simulink model "prach_shortFormat_fftShift"  (R2023b)
settings: Solver=FixedStepDiscrete  StartTime=0.0  StopTime=prach_short.SimulationTime  FixedStep=1  RelTol=1e-3  EnableMultiTasking=on
PreLoadFcn:
  | warning off Simulink:Commands:SetParamLinkChangeWarn
  | warning off Simulink:Commands:LoadMdlParameterizedLink
  | warning off Simulink:SL_SetParamLinkChangeWarn
  | warning off Simulink:SL_LoadMdlParameterizedLink
  | setup_prach_shortFormat;
InitFcn:
  | setup_prach_shortFormat;
StopFcn:
  | prach_post_run_script
values from neighbouring files (symbols this model uses):
  ConfigTable = [16 1 9,20,20,20,20,20,20,20,20,20 0 2 6 2 4 ... (first row only)    [ConfigIndexTable.m]
  NTxAnts = 4    [setup_prach_shortFormat.m]    (also in setup_prach_shortFormat_fftShift.m)
undefined symbols (not defined in the file or in its folder): AdvDSPBChannelOutDisplay, AdvDSPBDMemDisplay, BW, ControlDecode, display, dpoly, dspba, dspba_ChannelInVis, dspba_ChannelOutVis, dspba_internal_get_channel_ports, evalAionMaskParam, latency, PRACH_CC, PRACH_regs, prach_short, PrachLib, PrachLib_FFTshift, primtype, RemoveCP, Stream2BlockConv, UseDontCare, value, waveconfig
libraries: DSPBAPrim x397, DSPBAControl x16, DSPBAModelBus x7, DSPBABase x5, DSPBAUtilities x5, simulink x2, DSPBAVectorUtil x1, DspbAdvFftLibrary x1
(part 1 of 5)
Description:
  | This design Implements a PRACH detection for short format for TDD configurations.
settings Model: Creator=lrigby  LastModifiedBy=5g
settings SolverCC: AlgebraicLoopSolver=TrustRegion
settings DataIOCC: LimitDataPoints=on  SaveFormat=StructureWithTime  SignalLoggingSaveFormat=ModelDataLogs  ReturnWorkspaceOutputs=off
settings OptimizationCC: ExpressionDepthLimit=2147483647  InitFltsAndDblsToZero=on  LifeSpan=inf
settings DebuggingCC: SaveWithParameterizedLinksMsg=none  UnderspecifiedInitializationDetection=Classic  MergeDetectMultiDrivingBlocksExec=none  SignalResolutionControl=TryResolveAllWithWarning  SolverPrmCheckMsg=warning  ParameterPrecisionLossMsg=none  UnconnectedInputMsg=warning  UnconnectedOutputMsg=warning  UnconnectedLineMsg=warning  StateNameClashWarn=warning  SFUnexpectedBacktrackingDiag=warning  SFNoUnconditionalDefaultTransitionDiag=warning  SFExecutionAtInitializationDiag=none  ArithmeticOperatorsInVariantConditions=warning
settings HardwareCC: ProdBitPerPointer=32  ProdBitPerSizeT=32  ProdBitPerPtrDiffT=32  ProdLargestAtomicFloat=None  ProdIntDivRoundTo=Undefined  ProdEndianess=Unspecified  ProdWordSize=32  ProdHWDeviceType=ASIC/FPGA  TargetBitPerLong=64  TargetBitPerPointer=64  TargetBitPerSizeT=64  TargetBitPerPtrDiffT=64  TargetLongLongMode=on  TargetIntDivRoundTo=Zero  TargetEndianess=LittleEndian  TargetWordSize=64  TargetHWDeviceType=MATLAB Host  ProdEqTarget=off
settings ModelReferenceCC: EnableRefExpFcnMdlSchedulingChecks=on  PropagateSignalLabelsOutOfModel=off
settings SFSimCC: SimUseLocalCustomCode=off  SimParseCustomCode=off  CustomCodeUndefinedFunction=UseInterfaceOnly
settings RTWCC: RTWUseLocalCustomCode=off  DLArmComputeVersion=19.05
settings CodeAppCC: StateflowObjectComments=on
settings GRTTargetCC: TargetFcnLib=ansi_tfl_tmw.mat  TargetLangStandard=C89/C90 (ANSI)  CombineOutputUpdateFcns=off  GRTInterface=on
settings ConfigComp: CovMetricSettings=dw  CovSaveCumulativeToWorkspaceVar=on  CovSaveSingleToWorkspaceVar=on  CovExternalEMLEnable=off  CovSFcnEnable=off

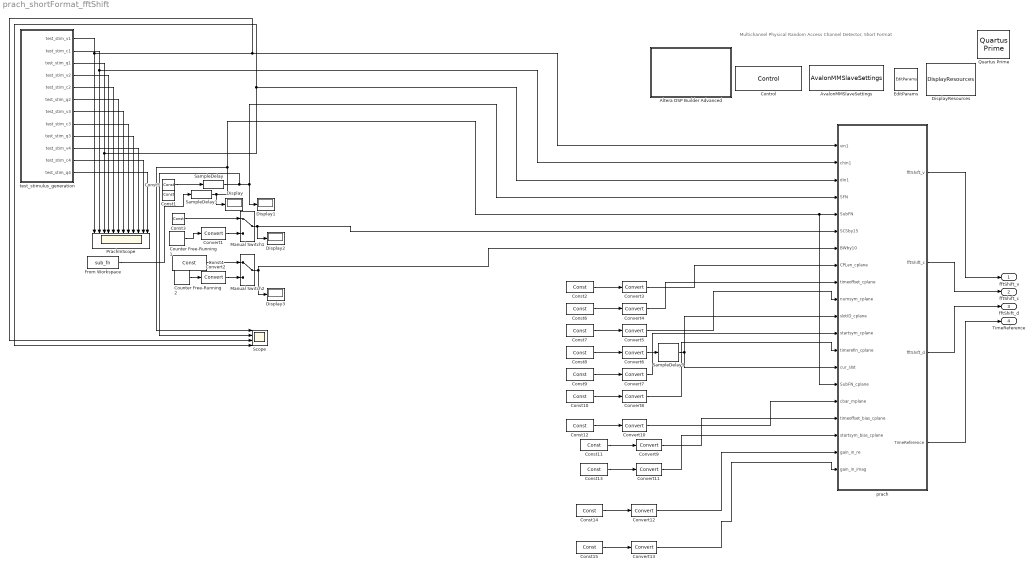
== system prach_shortFormat_fftShift ==
  note: Multichannel Physical Random
      | Access Channel Detector, Short Format
  Altera DSP Builder Advanced : Subsystem  mask(DSP Builder Advanced Blockset Ignored Block){}
      settings: OpenFcn=web('http://www.altera.com', '-new');
      mask Display: image(imread('alteralogo.tif'));
  AvalonMMSlaveSettings : DSPBABase/AvalonMMSlaveSettings
  Const1 : DSPBAPrim/Const  primtype=const  nInputs=0  nOutputs=1  omode=Specify via dialog  otype=uint(8)  scale=2^-0  rndmethod=Unbiased  factor=1  satmethod=Symmetric  shift_vec=[0 1 2 -1]  value=SubF  inPortNames=['+'; '+';]  outPortNames=[' ']  dspbaimage=dspba_prim.svg  text=fprintf('%s', num2str(value));  style=Optimised  visibilities=8 + 1024  floatPrecision=float32_m23  warnSaturation=on  version=20211007  SampleTime=inf
  Const{2,9..10,12..13,15} (6 alike) : DSPBAPrim/Const  primtype=const  nInputs=0  nOutputs=1  omode=Inherit via internal rule  otype=ufix(23)  scale=1  rndmethod=Unbiased  factor=1  satmethod=Symmetric  shift_vec=[0 1 2 -1]  value=0  inPortNames=['+'; '+';]  outPortNames=[' ']  dspbaimage=dspba_prim.svg  text=fprintf('%s', num2str(value));  style=Optimised  visibilities=8 + 1024  floatPrecision=float32_m23  warnSaturation=on  version=20211007  SampleTime=inf
  Const11 : DSPBAPrim/Const  primtype=const  nInputs=0  nOutputs=1  omode=Inherit via internal rule  otype=ufix(23)  scale=1  rndmethod=Unbiased  factor=1  satmethod=Symmetric  shift_vec=[0 1 2 -1]  value=220  inPortNames=['+'; '+';]  outPortNames=[' ']  dspbaimage=dspba_prim.svg  text=fprintf('%s', num2str(value));  style=Optimised  visibilities=8 + 1024  floatPrecision=float32_m23  warnSaturation=on  version=20211007  SampleTime=inf
  Const14 : DSPBAPrim/Const  primtype=const  nInputs=0  nOutputs=1  omode=Inherit via internal rule  otype=ufix(23)  scale=1  rndmethod=Unbiased  factor=1  satmethod=Symmetric  shift_vec=[0 1 2 -1]  value=1  inPortNames=['+'; '+';]  outPortNames=[' ']  dspbaimage=dspba_prim.svg  text=fprintf('%s', num2str(value));  style=Optimised  visibilities=8 + 1024  floatPrecision=float32_m23  warnSaturation=on  version=20211007  SampleTime=inf
  Const3 : DSPBAPrim/Const  primtype=const  nInputs=0  nOutputs=1  omode=Specify via dialog  otype=uint(2)  scale=1  rndmethod=Unbiased  factor=1  satmethod=Symmetric  shift_vec=[0 1 2 -1]  value=floor(waveconfig.PRACH.Config.SubcarrierSpacing/15)  inPortNames=['+'; '+';]  outPortNames=[' ']  dspbaimage=dspba_prim.svg  text=fprintf('%s', num2str(value));  style=Optimised  visibilities=8 + 1024  floatPrecision=float32_m23  warnSaturation=on  version=20211007  SampleTime=inf
  Const4 : DSPBAPrim/Const  primtype=const  nInputs=0  nOutputs=1  omode=Specify via dialog  otype=uint(4)  scale=1  rndmethod=Unbiased  factor=1  satmethod=Symmetric  shift_vec=[0 1 2 -1]  value=floor(BW/10)  inPortNames=['+'; '+';]  outPortNames=[' ']  dspbaimage=dspba_prim.svg  text=fprintf('%s', num2str(value));  style=Optimised  visibilities=8 + 1024  floatPrecision=float32_m23  warnSaturation=on  version=20211007  SampleTime=inf
  Const5 : DSPBAPrim/Const  primtype=const  nInputs=0  nOutputs=1  omode=Specify via dialog  otype=uint(12)  scale=2^-0  rndmethod=Unbiased  factor=1  satmethod=Symmetric  shift_vec=[0 1 2 -1]  value=SFN  inPortNames=['+'; '+';]  outPortNames=[' ']  dspbaimage=dspba_prim.svg  text=fprintf('%s', num2str(value));  style=Optimised  visibilities=8 + 1024  floatPrecision=float32_m23  warnSaturation=on  version=20211007  SampleTime=inf
  Const6 : DSPBAPrim/Const  primtype=const  nInputs=0  nOutputs=1  omode=Inherit via internal rule  otype=ufix(23)  scale=1  rndmethod=Unbiased  factor=1  satmethod=Symmetric  shift_vec=[0 1 2 -1]  value=1156  inPortNames=['+'; '+';]  outPortNames=[' ']  dspbaimage=dspba_prim.svg  text=fprintf('%s', num2str(value));  style=Optimised  visibilities=8 + 1024  floatPrecision=float32_m23  warnSaturation=on  version=20211007  SampleTime=inf
  Const7 : DSPBAPrim/Const  primtype=const  nInputs=0  nOutputs=1  omode=Inherit via internal rule  otype=ufix(23)  scale=1  rndmethod=Unbiased  factor=1  satmethod=Symmetric  shift_vec=[0 1 2 -1]  value=12  inPortNames=['+'; '+';]  outPortNames=[' ']  dspbaimage=dspba_prim.svg  text=fprintf('%s', num2str(value));  style=Optimised  visibilities=8 + 1024  floatPrecision=float32_m23  warnSaturation=on  version=20211007  SampleTime=inf
  Const8 : DSPBAPrim/Const  primtype=const  nInputs=0  nOutputs=1  omode=Inherit via internal rule  otype=ufix(23)  scale=1  rndmethod=Unbiased  factor=1  satmethod=Symmetric  shift_vec=[0 1 2 -1]  value=1  inPortNames=['+'; '+';]  outPortNames=[' ']  dspbaimage=dspba_prim.svg  text=fprintf('%s', num2str(value));  style=Optimised  visibilities=8 + 1024  floatPrecision=float32_m23  warnSaturation=on  version=20211007  SampleTime=inf
  Control : DSPBABase/Control  generate=on  language=VHDL  destination=./rtl  make_full_path=off  path_is_relative=on  autotestbench=on  signaldepth=2  coveragetestbench=off  logs=off  spacewidth=2  spacenum=1  addrwidth=10  datawidth=16  dataendian=Big Endian  hierarchicalnames=on  ramThresholdBits=-1  distRamThresholdBits=-1  mlabThresholdBits=-1  hardMultiplierThresholdLuts=-1  version=20090407  errorOnChanMismatch=1  errorOnGPIOMismatch=0  importModelsimResults=0  cycleAccurate=off  reinterpretCastMult=off  paramFile=prach_shortFormat_fftShift_params.xml
  Convert1 : DSPBAPrim/Convert  primtype=convert  nInputs=1  nOutputs=1  omode=Specify via dialog  otype=uint(2)  scale=1  rndmethod=Biased  factor=1  satmethod=None  shift_vec=[0 1 2 -1]  value=round([0:255]/17)  inPortNames=[' '; ' ';]  outPortNames=[' '; 'c']  dspbaimage=dspba_prim_wide.svg  text=fprintf('convert');  style=Optimised  visibilities=8+64+256+2^17  clipdetect=off  floatPrecision=float32_m23  advOptions=[]  version=20211007
  Convert10 : DSPBAPrim/Convert  primtype=convert  nInputs=1  nOutputs=1  omode=boolean  otype=ufix(2)  scale=1  rndmethod=Biased  factor=1  satmethod=None  shift_vec=[0 1 2 -1]  value=round([0:255]/17)  inPortNames=[' '; ' ';]  outPortNames=[' '; 'c']  dspbaimage=dspba_prim_wide.svg  text=fprintf('convert');  style=Optimised  visibilities=8+64+256+2^17  clipdetect=off  floatPrecision=float32_m23  advOptions=[]  version=20211007
  Convert{3..4,9,11} (4 alike) : DSPBAPrim/Convert  primtype=convert  nInputs=1  nOutputs=1  omode=Specify via dialog  otype=ufix(23)  scale=1  rndmethod=Biased  factor=1  satmethod=None  shift_vec=[0 1 2 -1]  value=round([0:255]/17)  inPortNames=[' '; ' ';]  outPortNames=[' '; 'c']  dspbaimage=dspba_prim_wide.svg  text=fprintf('convert');  style=Optimised  visibilities=8+64+256+2^17  clipdetect=off  floatPrecision=float32_m23  advOptions=[]  version=20211007
  Convert12 : DSPBAPrim/Convert  primtype=convert  nInputs=1  nOutputs=1  omode=Specify via dialog  otype=fixdt(0,16,14)  scale=0  rndmethod=Biased  factor=1  satmethod=None  shift_vec=[0 1 2 -1]  value=round([0:255]/17)  inPortNames=[' '; ' ';]  outPortNames=[' '; 'c']  dspbaimage=dspba_prim_wide.svg  text=fprintf('convert');  style=Optimised  visibilities=8+64+256+2^17  clipdetect=off  floatPrecision=float32_m23  advOptions=[]  version=20211007
  Convert13 : DSPBAPrim/Convert  primtype=convert  nInputs=1  nOutputs=1  omode=Specify via dialog  otype=fixdt(0,16,14)  scale=0  rndmethod=Biased  factor=1  satmethod=None  shift_vec=[0 1 2 -1]  value=round([0:255]/17)  inPortNames=[' '; ' ';]  outPortNames=[' '; 'c']  dspbaimage=dspba_prim_wide.svg  text=fprintf('convert');  style=Optimised  visibilities=8+64+256+2^17  clipdetect=off  floatPrecision=float32_m23  advOptions=[]  version=20211007
  Convert2 : DSPBAPrim/Convert  primtype=convert  nInputs=1  nOutputs=1  omode=Specify via dialog  otype=uint(8)  scale=1  rndmethod=Biased  factor=1  satmethod=None  shift_vec=[0 1 2 -1]  value=round([0:255]/17)  inPortNames=[' '; ' ';]  outPortNames=[' '; 'c']  dspbaimage=dspba_prim_wide.svg  text=fprintf('convert');  style=Optimised  visibilities=8+64+256+2^17  clipdetect=off  floatPrecision=float32_m23  advOptions=[]  version=20211007
  Convert5 : DSPBAPrim/Convert  primtype=convert  nInputs=1  nOutputs=1  omode=Specify via dialog  otype=ufix(4)  scale=1  rndmethod=Biased  factor=1  satmethod=None  shift_vec=[0 1 2 -1]  value=round([0:255]/17)  inPortNames=[' '; ' ';]  outPortNames=[' '; 'c']  dspbaimage=dspba_prim_wide.svg  text=fprintf('convert');  style=Optimised  visibilities=8+64+256+2^17  clipdetect=off  floatPrecision=float32_m23  advOptions=[]  version=20211007
  Convert6 : DSPBAPrim/Convert  primtype=convert  nInputs=1  nOutputs=1  omode=Specify via dialog  otype=ufix(2)  scale=1  rndmethod=Biased  factor=1  satmethod=None  shift_vec=[0 1 2 -1]  value=round([0:255]/17)  inPortNames=[' '; ' ';]  outPortNames=[' '; 'c']  dspbaimage=dspba_prim_wide.svg  text=fprintf('convert');  style=Optimised  visibilities=8+64+256+2^17  clipdetect=off  floatPrecision=float32_m23  advOptions=[]  version=20211007
  Convert7 : DSPBAPrim/Convert  primtype=convert  nInputs=1  nOutputs=1  omode=Specify via dialog  otype=ufix(4)  scale=1  rndmethod=Biased  factor=1  satmethod=None  shift_vec=[0 1 2 -1]  value=round([0:255]/17)  inPortNames=[' '; ' ';]  outPortNames=[' '; 'c']  dspbaimage=dspba_prim_wide.svg  text=fprintf('convert');  style=Optimised  visibilities=8+64+256+2^17  clipdetect=off  floatPrecision=float32_m23  advOptions=[]  version=20211007
  Convert8 : DSPBAPrim/Convert  primtype=convert  nInputs=1  nOutputs=1  omode=Specify via dialog  otype=ufix(29)  scale=1  rndmethod=Biased  factor=1  satmethod=None  shift_vec=[0 1 2 -1]  value=round([0:255]/17)  inPortNames=[' '; ' ';]  outPortNames=[' '; 'c']  dspbaimage=dspba_prim_wide.svg  text=fprintf('convert');  style=Optimised  visibilities=8+64+256+2^17  clipdetect=off  floatPrecision=float32_m23  advOptions=[]  version=20211007
  Counter Free-Running1 : simulink/Sources/Counter Free-Running  NumBits=2  tsamp=-1
  Counter Free-Running2 : simulink/Sources/Counter Free-Running  NumBits=4  tsamp=-1
  Display{,1..3} (4 alike) : Display
  DisplayResources : DSPBAUtilities/DisplayResources  mults=0  luts=0  memorybits=0
  EditParams : DSPBABase/EditParams  version=20090407
  From Workspace : FromWorkspace  VariableName=sub_fn  OutDataTypeStr=uint8  SampleTime=prach_short.SampleTime  OutputAfterFinalValue=Setting to zero
  Manual Switch1 : ManualSwitch
  Manual Switch2 : ManualSwitch
  PrachInScope : Scope  NumInputPorts=12
  Quartus Prime : DSPBABase/Quartus Prime  version=20090407
  SampleDelay : DSPBAPrim/SampleDelay  primtype=sampdelay  nInputs=1  nOutputs=1  omode=Inherit via internal rule  otype=sfix(16)  scale=2^-15  rndmethod=Unbiased  factor=1  satmethod=Symmetric  shift_vec=[0 1 2 -1]  floatPrecision=float32_m23  value=0  inPortNames=[' '; ' ';]  outPortNames=[' ']  dspbaimage=dspba_prim.svg  text=dpoly(1, eye(1,value+1), 'z')  style=Optimised  visibilities=8 + 1024 + 2^17 + 2^18  flexible=off  slackgroup=0  augmented=0  version=20211007  advOptions=[]
  SampleDelay1 : DSPBAPrim/SampleDelay  primtype=sampdelay  nInputs=1  nOutputs=1  omode=Inherit via internal rule  otype=sfix(16)  scale=2^-15  rndmethod=Unbiased  factor=1  satmethod=Symmetric  shift_vec=[0 1 2 -1]  floatPrecision=float32_m23  value=0  inPortNames=[' '; ' ';]  outPortNames=[' ']  dspbaimage=dspba_prim.svg  text=dpoly(1, eye(1,value+1), 'z')  style=Optimised  visibilities=8 + 1024 + 2^17 + 2^18  flexible=off  slackgroup=0  augmented=0  version=20211007  advOptions=[]
  SampleDelay5 : DSPBAPrim/SampleDelay  primtype=sampdelay  nInputs=1  nOutputs=1  omode=Inherit via internal rule  otype=sfix(16)  scale=2^-15  rndmethod=Unbiased  factor=1  satmethod=Symmetric  shift_vec=[0 1 2 -1]  floatPrecision=float32_m23  value=1  inPortNames=[' '; ' ';]  outPortNames=[' ']  dspbaimage=dspba_prim.svg  text=dpoly(1, eye(1,value+1), 'z')  style=Optimised  visibilities=8 + 1024 + 2^17 + 2^18  flexible=off  slackgroup=0  augmented=0  version=20211007  advOptions=[]
  Scope : Scope  NumInputPorts=4
  prach : Subsystem
  test_stimulus_generation : Subsystem
  fftShift_v : Outport
  fftShift_c : Outport  Port=2
  fftShift_d : Outport  Port=3
  TimeReference : Outport  Port=4
  wires:
  test_stimulus_generation/2(test_stim_c1) -> PrachInScope/2, prach/2(chin1)
  test_stimulus_generation/3(test_stim_q1) -> PrachInScope/3, Scope/4, prach/3(din1)
  test_stimulus_generation/4(test_stim_v2) -> PrachInScope/4
  test_stimulus_generation/5(test_stim_c2) -> PrachInScope/5
  test_stimulus_generation/6(test_stim_q2) -> PrachInScope/6
  test_stimulus_generation/7(test_stim_v3) -> PrachInScope/7
  test_stimulus_generation/8(test_stim_c3) -> PrachInScope/8
  test_stimulus_generation/9(test_stim_q3) -> PrachInScope/9
  test_stimulus_generation/10(test_stim_v4) -> PrachInScope/10
  test_stimulus_generation/11(test_stim_c4) -> PrachInScope/11
  test_stimulus_generation/12(test_stim_q4) -> PrachInScope/12
  test_stimulus_generation/1(test_stim_v1) -> PrachInScope/1, Scope/3, prach/1(vin1)
  Const5/1 -> SampleDelay/1
  From Workspace/1 -> SampleDelay1/1
  Const3/1 -> Manual Switch1/1
  Const4/1 -> Manual Switch2/1
  Manual Switch1/1 -> prach/6(SCSby15), Display2/1
  Manual Switch2/1 -> prach/7(BWby10), Display3/1
  Counter Free-Running1/1 -> Convert1/1
  Convert1/1 -> Manual Switch1/2
  Counter Free-Running2/1 -> Convert2/1
  Convert2/1 -> Manual Switch2/2
  SampleDelay/1 -> Scope/2, Display1/1, prach/4(SFN)
  SampleDelay1/1 -> Display/1, Scope/1, prach/15(SubFN_cplane), prach/5(SubFN)
  prach/3(fftShift_d) -> fftShift_d/1
  prach/2(fftShift_c) -> fftShift_c/1
  prach/4(TimeReference) -> TimeReference/1
  prach/1(fftShift_v) -> fftShift_v/1
  Const11/1 -> Convert9/1
  Convert9/1 -> prach/17(timeoffset_bias_cplane)
  Convert4/1 -> prach/9(timeoffset_cplane)
  Const8/1 -> Convert6/1
  Const10/1 -> Convert8/1
  Convert3/1 -> prach/8(CPLen_cplane)
  Const15/1 -> Convert13/1
  Const12/1 -> Convert10/1
  Convert5/1 -> prach/10(numsym_cplane)
  Const6/1 -> Convert4/1
  Convert7/1 -> prach/12(startsym_cplane)
  Convert8/1 -> prach/13(timerefin_cplane)
  Const7/1 -> Convert5/1
  Const2/1 -> Convert3/1
  Const9/1 -> Convert7/1
  Convert13/1 -> prach/20(gain_in_imag)
  Const13/1 -> Convert11/1
  Convert12/1 -> prach/19(gain_in_re)
  Convert11/1 -> prach/18(startsym_bias_cplane)
  Convert6/1 -> SampleDelay5/1
  SampleDelay5/1 -> prach/14(cur_slot), prach/11(slotID_cplane)
  Const14/1 -> Convert12/1
  Convert10/1 -> prach/16(cbar_mplane)

== system prach_shortFormat_fftShift/Altera DSP Builder Advanced ==

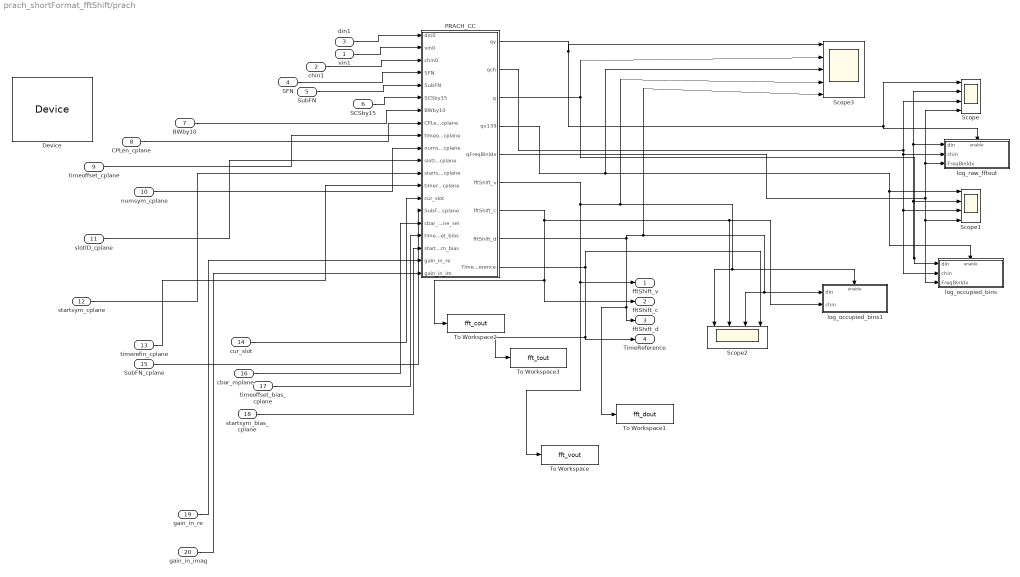
== system prach_shortFormat_fftShift/prach ==
  vin1 : Inport
  chin1 : Inport  Port=2
  din1 : Inport  Port=3
  SFN : Inport  Port=4
  SubFN : Inport  Port=5
  SCSby15 : Inport  Port=6
  BWby10 : Inport  Port=7
  CPLen_cplane : Inport  Port=8
  timeoffset_cplane : Inport  Port=9
  numsym_cplane : Inport  Port=10
  slotID_cplane : Inport  Port=11
  startsym_cplane : Inport  Port=12
  timerefin_cplane : Inport  Port=13
  cur_slot : Inport  Port=14
  SubFN_cplane : Inport  Port=15
  cbar_mplane : Inport  Port=16
  timeoffset_bias_cplane : Inport  Port=17
  startsym_bias_cplane : Inport  Port=18
  gain_in_re : Inport  Port=19
  gain_in_imag : Inport  Port=20
  Device : DSPBABase/Device  family=Arria 10  stratix4device=Stratix IV E  hardcopy4device=HardCopy IV E  stratix5device=Stratix V GX  device=AUTO  speed=1  stratixSpeed=-5  stratix2Speed=-3  stratix3Speed=-2  stratix4gxSpeed=-2  stratix4gtSpeed=-1  cyclone2Speed=-6  cyclone3Speed=-7  arria2Speed=-4  cyclone4eSpeed=-8  stratix5Speed=-3  arria5Speed=-4  arriaSpeed=-6  cyclone3lsSpeed=-7  cyclone5Speed=-6  arria2gzSpeed=-3  nightFurySpeed=-2  ecp2Speed=-7  hardcopycompat=off  version=20140217  max10flashmode=off  max10nomeminit=off
  PRACH_CC : Subsystem  AncestorBlock=PrachLib_FFTshift/PRACH_CC  mask{InstanceNumber=1}
      mask prompts: InstanceNumber "CC Index"
      mask init:
      | InstanceNumberStr = num2str(InstanceNumber)
      mask Display:
      | color('w');image('dspba_prim.jpg');
      | fprintf('Component\nCarrier\n\n %s\n\nPRACH', int2str(InstanceNumber));
      | port_label('input',1,'din');
      | port_label('input',2,'vin');
      | port_label('input',3,'chin');
      | port_label('input',4,'SFN');
      | port_label('input',5,'SubFN');
      | port_label('input',6,'SCS/15');
      | port_label('input',7,'BW/10');
      | port_label('output',1,'qv');
      | port_label('output',2,'qc');
      | port_label('output',3,'q');
      | port_label('output',4,'qv139');
      | port_label('output',5,'qFFTBinIdx');
  Scope : Scope  NumInputPorts=4
  Scope1 : Scope  NumInputPorts=4
  Scope2 : Scope  NumInputPorts=4
  Scope3 : Scope  NumInputPorts=5
  To Workspace : ToWorkspace  VariableName=fft_vout  SaveFormat=Timeseries  SampleTime=-1
  To Workspace1 : ToWorkspace  VariableName=fft_dout  SaveFormat=Timeseries  SampleTime=-1
  To Workspace2 : ToWorkspace  VariableName=fft_cout  SaveFormat=Timeseries  SampleTime=-1
  To Workspace3 : ToWorkspace  VariableName=fft_tout  SaveFormat=Timeseries  SampleTime=-1
  log_occupied_bins : Subsystem  TreatAsAtomicUnit=on
  log_occupied_bins1 : Subsystem  TreatAsAtomicUnit=on
  log_raw_fftout : Subsystem  TreatAsAtomicUnit=on
  fftShift_v : Outport
  fftShift_c : Outport  Port=2
  fftShift_d : Outport  Port=3
  TimeReference : Outport  Port=4
  wires:
  vin1/1 -> PRACH_CC/2(vin0)
  chin1/1 -> PRACH_CC/3(chin0)
  SFN/1 -> PRACH_CC/4(SFN)
  SubFN/1 -> PRACH_CC/5(SubFN)
  din1/1 -> PRACH_CC/1(din0)
  SCSby15/1 -> PRACH_CC/6(SCSby15)
  BWby10/1 -> PRACH_CC/7(BWby10)
  PRACH_CC/1(qv) -> log_raw_fftout/Enable, Scope/1, Scope3/1
  PRACH_CC/2(qch) -> Scope1/3, log_occupied_bins/2(chin), log_raw_fftout/2(chin), Scope/3
  PRACH_CC/3(q) -> log_occupied_bins/1(din), Scope1/2, Scope/2, log_raw_fftout/1(din), Scope3/2
  PRACH_CC/5(qFreqBinIdx) -> log_raw_fftout/3(FreqBinIdx), Scope/4, log_occupied_bins/3(FreqBinIdx), Scope1/4
  PRACH_CC/4(qv139) -> Scope3/3, log_occupied_bins/Enable, Scope1/1
  PRACH_CC/8(fftShift_d) -> fftShift_d/1, To Workspace1/1, Scope3/5, log_occupied_bins1/1(din), Scope2/3
  PRACH_CC/9(TimeReference) -> Scope2/4, To Workspace3/1, TimeReference/1
  PRACH_CC/6(fftShift_v) -> To Workspace/1, fftShift_v/1, Scope3/4, Scope2/1, log_occupied_bins1/Enable
  PRACH_CC/7(fftShift_c) -> To Workspace2/1, fftShift_c/1, log_occupied_bins1/2(chin), Scope2/2
  startsym_cplane/1 -> PRACH_CC/12(startsym_cplane)
  SubFN_cplane/1 -> PRACH_CC/15(SubFN_cplane)
  timeoffset_cplane/1 -> PRACH_CC/9(timeoffset_cplane)
  timeoffset_bias_cplane/1 -> PRACH_CC/17(time_offset_bias)
  CPLen_cplane/1 -> PRACH_CC/8(CPLen_cplane)
  gain_in_imag/1 -> PRACH_CC/20(gain_in_im)
  gain_in_re/1 -> PRACH_CC/19(gain_in_re)
  startsym_bias_cplane/1 -> PRACH_CC/18(startsym_bias)
  cbar_mplane/1 -> PRACH_CC/16(cbar_mplane_sel)
  timerefin_cplane/1 -> PRACH_CC/13(timerefin_cplane)
  slotID_cplane/1 -> PRACH_CC/11(slotID_cplane)
  cur_slot/1 -> PRACH_CC/14(cur_slot)
  numsym_cplane/1 -> PRACH_CC/10(numsym_cplane)

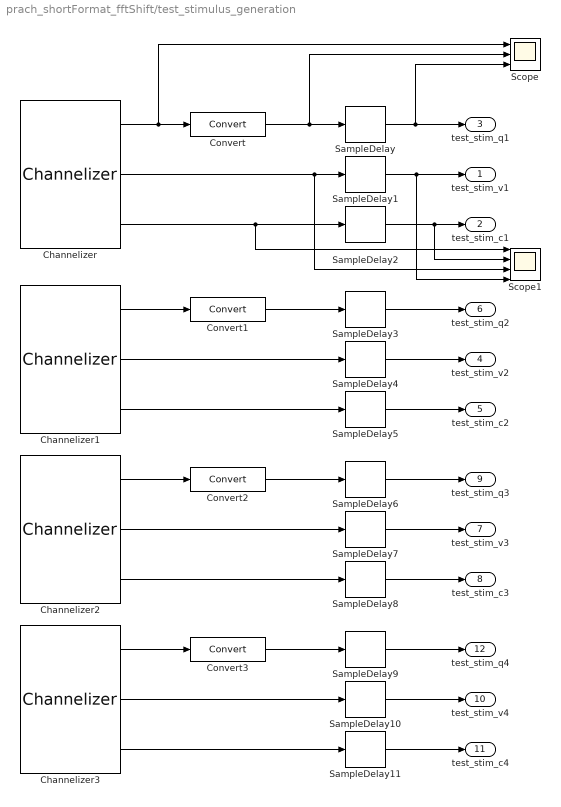
== system prach_shortFormat_fftShift/test_stimulus_generation ==
  Channelizer : DSPBAUtilities/Channelizer  data_input=prach_short.din  folding=prach_short.ClockRate/prach_short.SampleRateMSPS  samples_valid=NTxAnts  samples_idle=0  sample_time=prach_short.SampleTime
  Channelizer1 : DSPBAUtilities/Channelizer  data_input=prach_short.din  folding=prach_short.ClockRate/prach_short.SampleRateMSPS  samples_valid=NTxAnts  samples_idle=1  sample_time=prach_short.SampleTime
  Channelizer2 : DSPBAUtilities/Channelizer  data_input=prach_short.din  folding=prach_short.ClockRate/prach_short.SampleRateMSPS  samples_valid=NTxAnts  samples_idle=2  sample_time=prach_short.SampleTime
  Channelizer3 : DSPBAUtilities/Channelizer  data_input=-prach_short.din  folding=prach_short.ClockRate/prach_short.SampleRateMSPS  samples_valid=NTxAnts  samples_idle=3  sample_time=prach_short.SampleTime
  Convert{,1..3} (4 alike) : DSPBAPrim/Convert  primtype=convert  nInputs=1  nOutputs=1  omode=Specify via dialog  otype=sfix(16)  scale=2^-15  rndmethod=Biased  factor=1  satmethod=None  shift_vec=[0 1 2 -1]  value=round([0:255]/17)  inPortNames=[' '; ' ';]  outPortNames=[' '; 'c']  dspbaimage=dspba_prim_wide.svg  text=fprintf('convert');  style=Optimised  visibilities=8+64+256+2^17  clipdetect=off  floatPrecision=float32_m23  advOptions=[]  version=20211007
  SampleDelay{,1..6,8..9,11} (10 alike) : DSPBAPrim/SampleDelay  primtype=sampdelay  nInputs=1  nOutputs=1  omode=Inherit via internal rule  otype=sfix(16)  scale=2^-15  rndmethod=Unbiased  factor=1  satmethod=Symmetric  shift_vec=[0 1 2 -1]  floatPrecision=float32_m23  value=0  inPortNames=[' '; ' ';]  outPortNames=[' ']  dspbaimage=dspba_prim.svg  text=dpoly(1, eye(1,value+1), 'z')  style=Optimised  visibilities=8 + 1024 + 2^17 + 2^18  flexible=off  slackgroup=0  augmented=0  version=20211007  advOptions=[]
  SampleDelay10 : DSPBAPrim/SampleDelay  primtype=sampdelay  nInputs=1  nOutputs=1  omode=boolean  otype=sfix(16)  scale=2^-15  rndmethod=Unbiased  factor=1  satmethod=Symmetric  shift_vec=[0 1 2 -1]  floatPrecision=float32_m23  value=0  inPortNames=[' '; ' ';]  outPortNames=[' ']  dspbaimage=dspba_prim.svg  text=dpoly(1, eye(1,value+1), 'z')  style=Optimised  visibilities=8 + 1024 + 2^17 + 2^18  flexible=off  slackgroup=0  augmented=0  version=20211007  advOptions=[]
  SampleDelay7 : DSPBAPrim/SampleDelay  primtype=sampdelay  nInputs=1  nOutputs=1  omode=boolean  otype=sfix(16)  scale=2^-15  rndmethod=Unbiased  factor=1  satmethod=Symmetric  shift_vec=[0 1 2 -1]  floatPrecision=float32_m23  value=0  inPortNames=[' '; ' ';]  outPortNames=[' ']  dspbaimage=dspba_prim.svg  text=dpoly(1, eye(1,value+1), 'z')  style=Optimised  visibilities=8 + 1024 + 2^17 + 2^18  flexible=off  slackgroup=0  augmented=0  version=20211007  advOptions=[]
  Scope : Scope  NumInputPorts=3
  Scope1 : Scope  NumInputPorts=4
  test_stim_v1 : Outport  VectorParamsAs1DForOutWhenUnconnected=off
  test_stim_c1 : Outport  Port=2  VectorParamsAs1DForOutWhenUnconnected=off
  test_stim_q1 : Outport  Port=3  VectorParamsAs1DForOutWhenUnconnected=off
  test_stim_v2 : Outport  Port=4  VectorParamsAs1DForOutWhenUnconnected=off
  test_stim_c2 : Outport  Port=5  VectorParamsAs1DForOutWhenUnconnected=off
  test_stim_q2 : Outport  Port=6  VectorParamsAs1DForOutWhenUnconnected=off
  test_stim_v3 : Outport  Port=7  VectorParamsAs1DForOutWhenUnconnected=off
  test_stim_c3 : Outport  Port=8  VectorParamsAs1DForOutWhenUnconnected=off
  test_stim_q3 : Outport  Port=9  VectorParamsAs1DForOutWhenUnconnected=off
  test_stim_v4 : Outport  Port=10  VectorParamsAs1DForOutWhenUnconnected=off
  test_stim_c4 : Outport  Port=11  VectorParamsAs1DForOutWhenUnconnected=off
  test_stim_q4 : Outport  Port=12  VectorParamsAs1DForOutWhenUnconnected=off
  wires:
  Channelizer/1 -> Scope/1, Convert/1
  Convert/1 -> Scope/2, SampleDelay/1
  SampleDelay/1 -> Scope/3, test_stim_q1/1
  SampleDelay2/1 -> Scope1/2, test_stim_c1/1
  Channelizer/2 -> Scope1/3, SampleDelay1/1
  SampleDelay5/1 -> test_stim_c2/1
  SampleDelay3/1 -> test_stim_q2/1
  Channelizer1/3 -> SampleDelay5/1
  Channelizer1/2 -> SampleDelay4/1
  Convert1/1 -> SampleDelay3/1
  Channelizer1/1 -> Convert1/1
  SampleDelay8/1 -> test_stim_c3/1
  SampleDelay6/1 -> test_stim_q3/1
  Channelizer2/3 -> SampleDelay8/1
  Channelizer2/2 -> SampleDelay7/1
  Convert2/1 -> SampleDelay6/1
  Channelizer2/1 -> Convert2/1
  Channelizer3/2 -> SampleDelay10/1
  SampleDelay9/1 -> test_stim_q4/1
  Convert3/1 -> SampleDelay9/1
  Channelizer3/1 -> Convert3/1
  Channelizer3/3 -> SampleDelay11/1
  SampleDelay11/1 -> test_stim_c4/1
  SampleDelay4/1 -> test_stim_v2/1
  SampleDelay1/1 -> Scope1/4, test_stim_v1/1
  Channelizer/3 -> Scope1/1, SampleDelay2/1
  SampleDelay7/1 -> test_stim_v3/1
  SampleDelay10/1 -> test_stim_v4/1

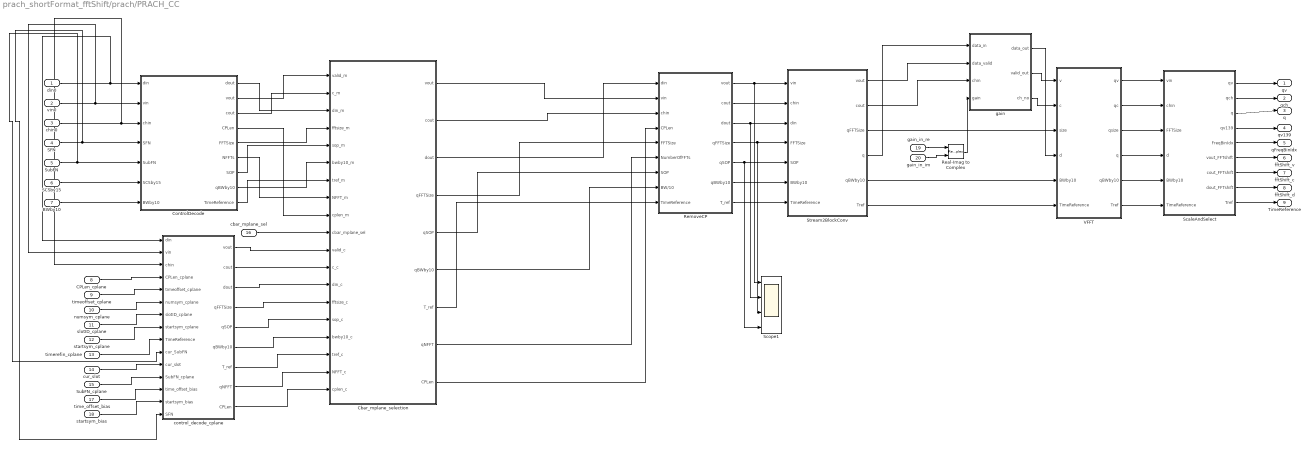
== system prach_shortFormat_fftShift/prach/PRACH_CC ==
  din0 : Inport
  vin0 : Inport  Port=2
  chin0 : Inport  Port=3
  SFN : Inport  Port=4
  SubFN : Inport  Port=5
  SCSby15 : Inport  Port=6
  BWby10 : Inport  Port=7
  CPLen_cplane : Inport  Port=8
  timeoffset_cplane : Inport  Port=9
  numsym_cplane : Inport  Port=10
  slotID_cplane : Inport  Port=11
  startsym_cplane : Inport  Port=12
  timerefin_cplane : Inport  Port=13
  cur_slot : Inport  Port=14
  SubFN_cplane : Inport  Port=15
  cbar_mplane_sel : Inport  Port=16
  time_offset_bias : Inport  Port=17
  startsym_bias : Inport  Port=18
  gain_in_re : Inport  Port=19
  gain_in_im : Inport  Port=20
  Cbar_mplane_selection : Subsystem
  ControlDecode : Subsystem  AncestorBlock=PrachLib/ControlDecode  mask{InstanceNumber=InstanceNumber}
      mask prompts: InstanceNumber "CC Index"
  Real-Imag to Complex : RealImagToComplex
  RemoveCP : Subsystem  AncestorBlock=PrachLib/RemoveCP  mask{NAnts=NTxAnts}
      mask prompts: NAnts "Number of Antennas"
  ScaleAndSelect : Subsystem
  Scope1 : Scope  NumInputPorts=4
  Stream2BlockConv : Subsystem  AncestorBlock=PrachLib/Stream2BlockConv  mask{NAnts=4, NFftMax=prach_short.Nfft}
      mask prompts: NAnts "Number of Antennas"; NFftMax "Maximum FFT size"
  VFFT : Subsystem  AncestorBlock=DspbAdvFftLibrary/Common/VFFT  Opaque=on  mask{IFFT=false, subchannels=1, br_in=true, maxSize=log2(prach_short.Nfft), minSize=9, in_type=prach_short.InputType, type_strings=prach_short.type_strings, faithful=false}
      mask prompts: subchannels "Number of interleaved subchannels (must be a power of 2)"; br_in "Bit-reversed input"; maxSize "maxSize, where the (I)FFT has at most 2^maxSize points"; minSize "minSize, where the (I)FFT has at least 2^minSize points"; in_type "Input type"; type_strings "Twiddle/pruning specification"; faithful "Use faithful rounding"
      mask init:
      | block = gcb;
      | 
      | % Check that we have a legal number of subchannels
      | subchannelbits = ceil(log2(subchannels));
      | if not(subchannels == 2^subchannelbits)
      |     error('%s: subchannels count %d is not a power of 2', block, subchannels);
      | end
      | 
      | if IFFT
      |     FFTstring = 'IFFT';
      | else
      |     FFTstring = 'FFT';
      | end
      | 
      | if br_in
      |     directionString = 'BR->NAT';
      | else
      |     directionString = 'NAT->BR';
      | end
      | 
      | if 1 < subchannels
      |     subchannelString = sprintf('%d subchannels',subchannels);
      | else
      |     subchannelString = '';
      | end
      mask Help: helpview(dspba.GetHelp('fft'));
      mask Display:
      | color('w');
      | image('dspba_fft.jpg');
      | port_label('input',1,'v');
      | port_label('input',2,'c');
      | port_label('input',3,'size');
      | port_label('input',4,'d');
      | port_label('input',5,'BW/10');
      | port_label('output',1,'qv');
      | port_label('output',2,'qc');
      | port_label('output',3,'qsize');
      | port_label('output',4,'q');
      | port_label('output',5,'qBW/10');
      | text(0.30,0.65,sprintf('V%s Core',FFTstring));
      | text(0.35,0.55,sprintf('2^{%d} to 2^{%d}',minSize,maxSize),'texmode','on');
      | text(0.30,0.45,directionString);
      | text(0.20,0.30,subchannelString);
  control_decode_cplane : Subsystem
  gain : Subsystem
  qv : Outport
  qch : Outport  Port=2
  q : Outport  Port=3
  qv139 : Outport  Port=4
  qFreqBinIdx : Outport  Port=5
  fftShift_v : Outport  Port=6
  fftShift_c : Outport  Port=7
  fftShift_d : Outport  Port=8
  TimeReference : Outport  Port=9
  wires:
  Stream2BlockConv/4(q) -> gain/1(data_in)
  Stream2BlockConv/3(qFFTSize) -> VFFT/3(size)
  Stream2BlockConv/2(cout) -> gain/3(chin)
  Stream2BlockConv/1(vout) -> gain/2(data_valid)
  VFFT/5(qBWby10) -> ScaleAndSelect/5(BWby10)
  Stream2BlockConv/5(qBWby10) -> VFFT/5(BWby10)
  RemoveCP/6(qBWby10) -> Stream2BlockConv/6(BWby10)
  ScaleAndSelect/5(FreqBinIdx) -> qFreqBinIdx/1
  ScaleAndSelect/4(qv139) -> qv139/1
  ScaleAndSelect/3(q) -> q/1
  ScaleAndSelect/2(qch) -> qch/1
  ScaleAndSelect/1(qv) -> qv/1
  VFFT/4(q) -> ScaleAndSelect/4(d)
  VFFT/3(qsize) -> ScaleAndSelect/3(FFTSize)
  VFFT/2(qc) -> ScaleAndSelect/2(chin)
  VFFT/1(qv) -> ScaleAndSelect/1(vin)
  RemoveCP/5(qSOP) -> Scope1/4, Stream2BlockConv/5(SOP)
  RemoveCP/4(qFFTSize) -> Scope1/3, Stream2BlockConv/4(FFTSize)
  RemoveCP/3(dout) -> Stream2BlockConv/3(din), Scope1/2
  RemoveCP/1(vout) -> Stream2BlockConv/1(vin), Scope1/1
  RemoveCP/2(cout) -> Stream2BlockConv/2(chin)
  SCSby15/1 -> ControlDecode/6(SCSby15)
  BWby10/1 -> ControlDecode/7(BWby10)
  vin0/1 -> control_decode_cplane/2(vin), ControlDecode/2(vin)
  chin0/1 -> control_decode_cplane/3(chin), ControlDecode/3(chin)
  SubFN/1 -> control_decode_cplane/10(cur_SubFN), ControlDecode/5(SubFN)
  din0/1 -> control_decode_cplane/1(din), ControlDecode/1(din)
  SFN/1 -> control_decode_cplane/15(SFN), ControlDecode/4(SFN)
  ScaleAndSelect/7(cout_FFTshift) -> fftShift_c/1
  ScaleAndSelect/8(dout_FFTshift) -> fftShift_d/1
  ScaleAndSelect/6(vout_FFTshift) -> fftShift_v/1
  RemoveCP/7(T_ref) -> Stream2BlockConv/7(TimeReference)
  Stream2BlockConv/6(Tref) -> VFFT/6(TimeReference)
  VFFT/6(Tref) -> ScaleAndSelect/6(TimeReference)
  ScaleAndSelect/9(Tref) -> TimeReference/1
  SubFN_cplane/1 -> control_decode_cplane/12(SubFN_cplane)
  control_decode_cplane/1(vout) -> Cbar_mplane_selection/11(valid_c)
  CPLen_cplane/1 -> control_decode_cplane/4(CPLen_cplane)
  startsym_bias/1 -> control_decode_cplane/14(startsym_bias)
  control_decode_cplane/9(CPLen) -> Cbar_mplane_selection/19(cplen_c)
  timerefin_cplane/1 -> control_decode_cplane/9(TimeReference)
  timeoffset_cplane/1 -> control_decode_cplane/5(timeoffset_cplane)
  control_decode_cplane/5(qSOP) -> Cbar_mplane_selection/15(sop_c)
  control_decode_cplane/2(cout) -> Cbar_mplane_selection/12(c_c)
  control_decode_cplane/8(qNFFT) -> Cbar_mplane_selection/18(NFFT_c)
  control_decode_cplane/3(dout) -> Cbar_mplane_selection/13(din_c)
  control_decode_cplane/7(T_ref) -> Cbar_mplane_selection/17(tref_c)
  startsym_cplane/1 -> control_decode_cplane/8(startsym_cplane)
  slotID_cplane/1 -> control_decode_cplane/7(slotID_cplane)
  time_offset_bias/1 -> control_decode_cplane/13(time_offset_bias)
  numsym_cplane/1 -> control_decode_cplane/6(numsym_cplane)
  control_decode_cplane/6(qBWby10) -> Cbar_mplane_selection/16(bwby10_c)
  cbar_mplane_sel/1 -> Cbar_mplane_selection/10(cbar_mplane_sel)
  cur_slot/1 -> control_decode_cplane/11(cur_slot)
  control_decode_cplane/4(qFFTSize) -> Cbar_mplane_selection/14(fftsize_c)
  ControlDecode/2(vout) -> Cbar_mplane_selection/1(valid_m)
  ControlDecode/1(dout) -> Cbar_mplane_selection/3(din_m)
  ControlDecode/3(cout) -> Cbar_mplane_selection/2(c_m)
  ControlDecode/4(CPLen) -> Cbar_mplane_selection/9(cplen_m)
  ControlDecode/5(FFTSize) -> Cbar_mplane_selection/4(fftsize_m)
  ControlDecode/6(NFFTs) -> Cbar_mplane_selection/8(NFFT_m)
  ControlDecode/7(SOP) -> Cbar_mplane_selection/5(sop_m)
  ControlDecode/8(qBWby10) -> Cbar_mplane_selection/6(bwby10_m)
  ControlDecode/9(TimeReference) -> Cbar_mplane_selection/7(tref_m)
  Cbar_mplane_selection/1(vout) -> RemoveCP/2(vin)
  Cbar_mplane_selection/2(cout) -> RemoveCP/3(chin)
  Cbar_mplane_selection/3(dout) -> RemoveCP/1(din)
  Cbar_mplane_selection/4(qFFTSize) -> RemoveCP/5(FFTSize)
  Cbar_mplane_selection/5(qSOP) -> RemoveCP/7(SOP)
  Cbar_mplane_selection/6(qBWby10) -> RemoveCP/8(BW/10)
  Cbar_mplane_selection/7(T_ref) -> RemoveCP/9(TimeReference)
  Cbar_mplane_selection/8(qNFFT) -> RemoveCP/6(NumberOfFFTs)
  Cbar_mplane_selection/9(CPLen) -> RemoveCP/4(CPLen)
  gain/1(data_out) -> VFFT/4(d)
  gain/2(valid_out) -> VFFT/1(v)
  gain/3(ch_no) -> VFFT/2(c)
  gain_in_re/1 -> Real-Imag to Complex/1
  gain_in_im/1 -> Real-Imag to Complex/2
  Real-Imag to Complex/1 -> gain/4(gain)

== system prach_shortFormat_fftShift/prach/log_occupied_bins ==
  din : Inport
  chin : Inport  Port=2
  FreqBinIdx : Inport  Port=3
  Enable : EnablePort
  To Workspace : ToWorkspace  VariableName=PrachOut139_DSPBA  SampleTime=-1
  To Workspace1 : ToWorkspace  VariableName=PrachIdxOut139_DSPBA  SampleTime=-1
  To Workspace2 : ToWorkspace  VariableName=PrachAntOut139_DSPBA  SampleTime=-1
  wires:
  chin/1 -> To Workspace2/1
  din/1 -> To Workspace/1
  FreqBinIdx/1 -> To Workspace1/1

== system prach_shortFormat_fftShift/prach/log_occupied_bins1 ==
  din : Inport
  chin : Inport  Port=2
  Enable : EnablePort
  To Workspace : ToWorkspace  VariableName=PrachOut139_fftShift  SampleTime=-1
      settings: Save2DSignal=2-D array (concatenate along first dimension)
  To Workspace2 : ToWorkspace  VariableName=PrachAntOut139_fftShift  SampleTime=-1
  wires:
  din/1 -> To Workspace/1
  chin/1 -> To Workspace2/1

== system prach_shortFormat_fftShift/prach/log_raw_fftout ==
  din : Inport
  chin : Inport  Port=2
  FreqBinIdx : Inport  Port=3
  Enable : EnablePort
  To Workspace : ToWorkspace  VariableName=PrachOut_DSPBA  SampleTime=-1
  To Workspace1 : ToWorkspace  VariableName=PrachIdxOut_DSPBA  SampleTime=-1
  To Workspace2 : ToWorkspace  VariableName=PrachAntOut_DSPBA  SampleTime=-1
  wires:
  FreqBinIdx/1 -> To Workspace1/1
  din/1 -> To Workspace/1
  chin/1 -> To Workspace2/1

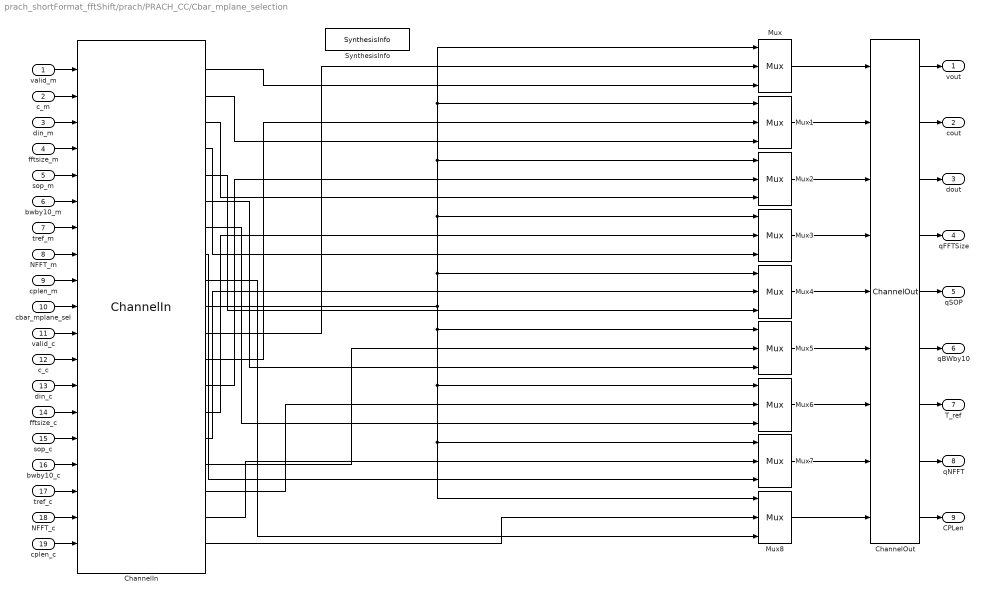
== system prach_shortFormat_fftShift/prach/PRACH_CC/Cbar_mplane_selection ==
  valid_m : Inport
  c_m : Inport  Port=2
  din_m : Inport  Port=3
  fftsize_m : Inport  Port=4
  sop_m : Inport  Port=5
  bwby10_m : Inport  Port=6
  tref_m : Inport  Port=7
  NFFT_m : Inport  Port=8
  cplen_m : Inport  Port=9
  cbar_mplane_sel : Inport  Port=10
  valid_c : Inport  Port=11
  c_c : Inport  Port=12
  din_c : Inport  Port=13
  fftsize_c : Inport  Port=14
  sop_c : Inport  Port=15
  bwby10_c : Inport  Port=16
  tref_c : Inport  Port=17
  NFFT_c : Inport  Port=18
  cplen_c : Inport  Port=19
  ChannelIn : DSPBAPrim/ChannelIn  primtype=channelin  nInputs=dspba_internal_get_channel_ports(gcb)  nOutputs=dspba_internal_get_channel_ports(gcb)  omode=Inherit via internal rule  otype=sfix(16)  scale=2^-15  rndmethod=Unbiased  factor=1  satmethod=Symmetric  shift_vec=[0 1 2 -1]  value=17  inPortNames=['v'; 'c'; '0'; '1'; '2'; '3'; '4'; '5'; '6'; '7'; '8'; '9'; 'A'; 'B'; 'D'; 'E'; 'F'; 'G'; 'H'; 'I'; 'J'; 'K'; 'L'; 'M'; 'N'; 'O'; 'P'; 'Q'; 'R'; 'S'; 'T'; 'U'; 'W'; 'X'; 'Y'; 'Z']  outPortNames=['v'; 'c'; '0'; '1'; '2'; '3'; '4'; '5'; '6'; '7'; '8'; '9'; 'A'; 'B'; 'D'; 'E'; 'F'; 'G'; 'H'; 'I'; 'J'; 'K'; 'L'; 'M'; 'N'; 'O'; 'P'; 'Q'; 'R'; 'S'; 'T'; 'U'; 'W'; 'X'; 'Y'; 'Z']  dspbaimage=dspba_prim_channel_tall.svg  text=fprintf('In');  style=Optimised  dataSignals=17  foldingEnabled=off  channels=1  sampleRate=200  packetBeginPresent=off  packetBeginEnabled=off  visibilities=dspba_ChannelInVis(gcb)  scheduleOrigin=on  version=20211214
  ChannelOut : DSPBAPrim/ChannelOut  primtype=channelout  nInputs=dspba_internal_get_channel_ports(gcb)  nOutputs=dspba_internal_get_channel_ports(gcb)  omode=Inherit via internal rule  otype=sfix(16)  scale=2^-15  rndmethod=Unbiased  factor=1  satmethod=Symmetric  shift_vec=[0 1 2 -1]  value=7  inPortNames=['v'; 'c'; '0'; '1'; '2'; '3'; '4'; '5'; '6'; '7'; '8'; '9'; 'A'; 'B'; 'D'; 'E'; 'F'; 'G'; 'H'; 'I'; 'J'; 'K'; 'L'; 'M'; 'N'; 'O'; 'P'; 'Q'; 'R'; 'S'; 'T'; 'U'; 'W'; 'X'; 'Y'; 'Z']  outPortNames=['v'; 'c'; '0'; '1'; '2'; '3'; '4'; '5'; '6'; '7'; '8'; '9'; 'A'; 'B'; 'D'; 'E'; 'F'; 'G'; 'H'; 'I'; 'J'; 'K'; 'L'; 'M'; 'N'; 'O'; 'P'; 'Q'; 'R'; 'S'; 'T'; 'U'; 'W'; 'X'; 'Y'; 'Z']  dspbaimage=dspba_prim_channel_tall.svg  text=fprintf('Out%s', AdvDSPBChannelOutDisplay(latency));  style=Optimised  dataSignals=7  foldingEnabled=off  channels=1  sampleRate=200  packetBeginPresent=off  packetBeginEnabled=off  visibilities=dspba_ChannelOutVis(gcb)  latency=1  version=20211214
  Mux{,1..8} (9 alike) : DSPBAPrim/Mux  primtype=mux  nInputs=evalAionMaskParam(gcb,'value',1)+1  nOutputs=1  omode=Inherit via internal rule  otype=sfix(16)  scale=2^-15  rndmethod=Unbiased  factor=1  satmethod=Symmetric  shift_vec=[0 1 2 -1]  value=2  inPortNames=['s '; 'd0'; 'd1'; 'd2'; 'd3'; 'd4'; 'd5'; 'd6'; 'd7'; 'd8'; 'd9';]  outPortNames=[' ']  dspbaimage=dspba_prim_tall.svg  text=fprintf('%s', primtype);  style=Optimised  visibilities=1032  version=20211007
  SynthesisInfo : DSPBAPrim/SynthesisInfo  primtype=synthinfo  nInputs=0  nOutputs=0  omode=Inherit via internal rule  otype=sfix(16)  scale=2^-15  rndmethod=Truncate  factor=1  satmethod=Symmetric  shift_vec=[0 1 2 -1]  value=99  inPortNames=[' '; ' ';]  outPortNames=[' ']  dspbaimage=dspba_prim_ctrl.jpg  text=fprintf('Style=%s', style);  style=Scheduled  visibilities=2^17+2^18+2^19+2^20+2^21+2^22+2^23+2^24  constraintPair=None  constraintRelation=>  constraintLimit=6  modelRefSign=+  modelRef=''  showSchedule=off  simulationMode=Use Global Value  resetMinimization=Conditional - On for ChannelIn/Out only  version=20220106
  vout : Outport  VectorParamsAs1DForOutWhenUnconnected=off
  cout : Outport  Port=2  VectorParamsAs1DForOutWhenUnconnected=off
  dout : Outport  Port=3  VectorParamsAs1DForOutWhenUnconnected=off
  qFFTSize : Outport  Port=4  VectorParamsAs1DForOutWhenUnconnected=off
  qSOP : Outport  Port=5  VectorParamsAs1DForOutWhenUnconnected=off
  qBWby10 : Outport  Port=6  VectorParamsAs1DForOutWhenUnconnected=off
  T_ref : Outport  Port=7  VectorParamsAs1DForOutWhenUnconnected=off
  qNFFT : Outport  Port=8
  CPLen : Outport  Port=9
  wires:
  cplen_c/1 -> ChannelIn/19
  NFFT_c/1 -> ChannelIn/18
  bwby10_c/1 -> ChannelIn/16
  c_c/1 -> ChannelIn/12
  valid_c/1 -> ChannelIn/11
  cbar_mplane_sel/1 -> ChannelIn/10
  NFFT_m/1 -> ChannelIn/8
  fftsize_c/1 -> ChannelIn/14
  tref_m/1 -> ChannelIn/7
  bwby10_m/1 -> ChannelIn/6
  tref_c/1 -> ChannelIn/17
  ChannelOut/1 -> vout/1
  sop_c/1 -> ChannelIn/15
  ChannelOut/9 -> CPLen/1
  ChannelOut/5 -> qSOP/1
  ChannelOut/6 -> qBWby10/1
  ChannelOut/7 -> T_ref/1
  din_c/1 -> ChannelIn/13
  sop_m/1 -> ChannelIn/5
  ChannelOut/4 -> qFFTSize/1
  ChannelOut/8 -> qNFFT/1
  cplen_m/1 -> ChannelIn/9
  ChannelOut/2 -> cout/1
  c_m/1 -> ChannelIn/2
  din_m/1 -> ChannelIn/3
  ChannelOut/3 -> dout/1
  valid_m/1 -> ChannelIn/1
  fftsize_m/1 -> ChannelIn/4
  ChannelIn/10 -> Mux8/1, Mux7/1, Mux6/1, Mux5/1, Mux3/1, Mux1/1, Mux/1, Mux2/1, Mux4/1
  Mux/1 -> ChannelOut/1
  Mux1/1 -> ChannelOut/2
  Mux2/1 -> ChannelOut/3
  Mux3/1 -> ChannelOut/4
  Mux4/1 -> ChannelOut/5
  Mux5/1 -> ChannelOut/6
  Mux6/1 -> ChannelOut/7
  Mux7/1 -> ChannelOut/8
  Mux8/1 -> ChannelOut/9
  ChannelIn/11 -> Mux/2
  ChannelIn/12 -> Mux1/2
  ChannelIn/13 -> Mux2/2
  ChannelIn/14 -> Mux3/2
  ChannelIn/15 -> Mux4/2
  ChannelIn/16 -> Mux5/2
  ChannelIn/17 -> Mux6/2
  ChannelIn/18 -> Mux7/2
  ChannelIn/19 -> Mux8/2
  ChannelIn/1 -> Mux/3
  ChannelIn/2 -> Mux1/3
  ChannelIn/3 -> Mux2/3
  ChannelIn/4 -> Mux3/3
  ChannelIn/5 -> Mux4/3
  ChannelIn/6 -> Mux5/3
  ChannelIn/7 -> Mux6/3
  ChannelIn/8 -> Mux7/3
  ChannelIn/9 -> Mux8/3
